simulink model "MAIN_Submitted_to_UMD_V2_PCLC_Sim_Hem"  (R2024a)
settings: Solver=ode3  StartTime=0.0  StopTime=T_end  FixedStep=0.01  RelTol=1e-3  EnableMultiTasking=on
values from neighbouring files (symbols this model uses):
  A1 = x(1)    [MAIN_Protocol_Simulation.m]    (also in find_fluid_profile.m)
  A2 = x(2)    [MAIN_Protocol_Simulation.m]    (also in find_fluid_profile.m)
  A3 = x(8)    [MAIN_Protocol_Simulation.m]    (also in find_fluid_profile.m)
  A4 = x(12)    [MAIN_Protocol_Simulation.m]    (also in find_fluid_profile.m)
  B_Gain = x(3)    [MAIN_Protocol_Simulation.m]    (also in find_fluid_profile.m)
  B_Loss = x(4)    [MAIN_Protocol_Simulation.m]    (also in find_fluid_profile.m)
  BP_Tar = x(14)    [MAIN_Protocol_Simulation.m]    (also in find_fluid_profile.m)
  BV0 = x(25)    [MAIN_Protocol_Simulation.m]    (also in find_fluid_profile.m)
  G1 = x(15)    [MAIN_Protocol_Simulation.m]    (also in find_fluid_profile.m)
  G2 = x(16)    [MAIN_Protocol_Simulation.m]    (also in find_fluid_profile.m)
  G3 = x(19)    [MAIN_Protocol_Simulation.m]    (also in find_fluid_profile.m)
  gap_btn_hem = 0.5    [find_fluid_profile.m]
  Gsv1 = x(6)    [MAIN_Protocol_Simulation.m]    (also in find_fluid_profile.m)
  Gsv2 = x(7)    [MAIN_Protocol_Simulation.m]    (also in find_fluid_profile.m)
  H = (0.04022*W-0.1436)/60    [find_fluid_profile.m]
  Hct0 = x(24)    [MAIN_Protocol_Simulation.m]    (also in find_fluid_profile.m)
  HR0 = x(22)    [MAIN_Protocol_Simulation.m]    (also in find_fluid_profile.m)
  Ki4 = x(21)    [MAIN_Protocol_Simulation.m]    (also in find_fluid_profile.m)
  Kp = x(5)    [MAIN_Protocol_Simulation.m]    (also in find_fluid_profile.m)
  Kp2 = x(10)    [MAIN_Protocol_Simulation.m]    (also in find_fluid_profile.m)
  Kp3 = x(11)    [MAIN_Protocol_Simulation.m]    (also in find_fluid_profile.m)
  Kp4 = x(20)    [MAIN_Protocol_Simulation.m]    (also in find_fluid_profile.m)
  maintain_time = 15    [find_fluid_profile.m]
  max_hem_time = 1    [find_fluid_profile.m]
  max_sim_time = 120    [find_fluid_profile.m]
  pow1 = x(17)    [MAIN_Protocol_Simulation.m]    (also in find_fluid_profile.m)
  pow2 = x(18)    [MAIN_Protocol_Simulation.m]    (also in find_fluid_profile.m)
  SV0 = x(23)    [MAIN_Protocol_Simulation.m]    (also in find_fluid_profile.m = theta_s(18))
  SV_Tar = x(9)    [MAIN_Protocol_Simulation.m]    (also in find_fluid_profile.m)
  TPR0 = x(13)    [MAIN_Protocol_Simulation.m]    (also in find_fluid_profile.m)
libraries: simulink x1
settings Model: Creator=Ramin  LastModifiedBy=yekanth
settings SolverCC: AlgebraicLoopSolver=TrustRegion
settings DataIOCC: LimitDataPoints=on  SaveFormat=Array  SignalLoggingSaveFormat=ModelDataLogs  ReturnWorkspaceOutputs=off
settings OptimizationCC: ExpressionDepthLimit=2147483647  LifeSpan=inf
settings DebuggingCC: UnderspecifiedInitializationDetection=Classic  MergeDetectMultiDrivingBlocksExec=none  SolverPrmCheckMsg=warning  FcnCallInpInsideContextMsg=warning  UnconnectedInputMsg=warning  UnconnectedOutputMsg=warning  UnconnectedLineMsg=warning  StateNameClashWarn=warning  SFUnexpectedBacktrackingDiag=warning  SFNoUnconditionalDefaultTransitionDiag=warning  SFExecutionAtInitializationDiag=none  ArithmeticOperatorsInVariantConditions=warning
settings HardwareCC: ProdBitPerPointer=32  ProdBitPerSizeT=32  ProdBitPerPtrDiffT=32  ProdLargestAtomicFloat=None  ProdIntDivRoundTo=Undefined  ProdEndianess=Unspecified  ProdWordSize=32  ProdHWDeviceType=32-bit Generic
settings ModelReferenceCC: EnableRefExpFcnMdlSchedulingChecks=on  PropagateSignalLabelsOutOfModel=off
settings SFSimCC: SimUseLocalCustomCode=off  LegacyBehaviorForPersistentVarInContinuousTime=on  CustomCodeUndefinedFunction=UseInterfaceOnly
settings RTWCC: RTWUseLocalCustomCode=off  GPUComputeCapability=3.5
settings CodeAppCC: StateflowObjectComments=on
settings GRTTargetCC: TargetLangStandard=C89/C90 (ANSI)
settings ConfigComp: CovMetricSettings=dw  CovSaveCumulativeToWorkspaceVar=on  CovSaveSingleToWorkspaceVar=on  CovExternalEMLEnable=off

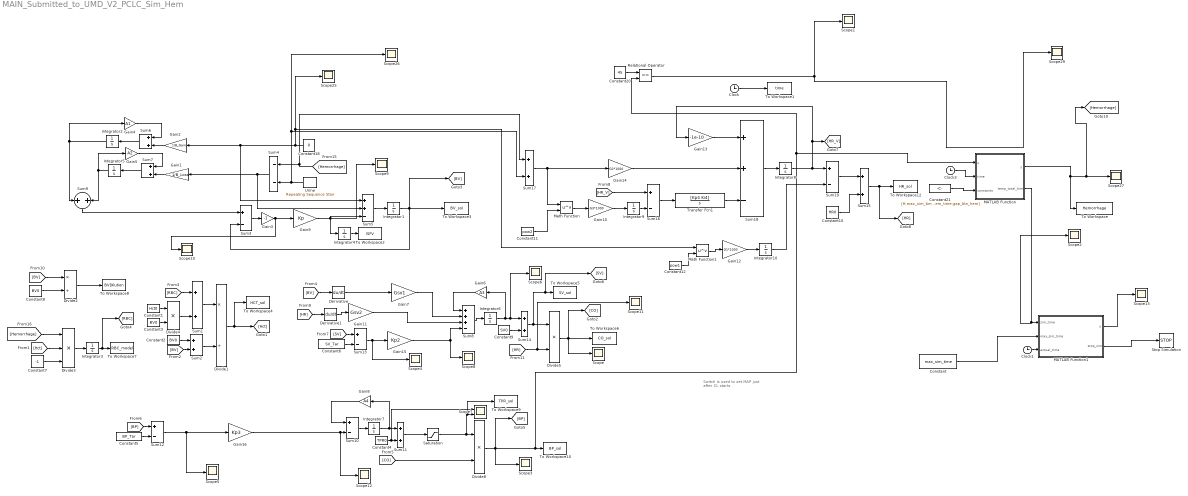
== system MAIN_Submitted_to_UMD_V2_PCLC_Sim_Hem ==
  note: Switch is used to set MAP just
      |  after CL starts
  Clock : Clock
  Clock1 : Clock
  Clock3 : Clock
  Constant : Constant  Value=max_sim_time
  Constant1 : Constant  Value=Hct0
  Constant10 : Constant  Value=HR0
  Constant11 : Constant  Value=pow2
  Constant12 : Constant  Value=pow1
  Constant18 : Constant  Value=0
  Constant2 : Constant  Value=BV0
  Constant20 : Constant  Value=45
  Constant21 : Constant  Value=[H;max_sim_time;maintain_time;max_hem_time;gap_btn_hem]  VectorParams1D=off
  Constant3 : Constant  Value=BV0
  Constant4 : Constant  Value=TPR0
  Constant5 : Constant  Value=BP_Tar
  Constant6 : Constant  Value=SV_Tar
  Constant7 : Constant  Value=-1
  Constant8 : Constant  Value=BV0
  Constant9 : Constant  Value=SV0
  Derivative : Derivative
  Derivative1 : Derivative
  Divide1 : Product  Inputs=*/
  Divide2 : Product  Inputs=*/
  Divide3 : Product  Inputs=***
  Divide4 : Product  Inputs=**
  Divide5 : Product  Inputs=**
  Divide8 : Product  Inputs=**
  Gain1 : Gain  Gain=1/B_Loss
  Gain10 : Gain  Gain=G3*1000
  Gain11 : Gain  Gain=Gsv2
  Gain12 : Gain  Gain=G1*1000
  Gain13 : Gain  Gain=-1e-10
  Gain14 : Gain  Gain=G2*1000
  Gain15 : Gain  Gain=Kp2
  Gain16 : Gain  Gain=Kp3
  Gain2 : Gain  Gain=1/B_Gain
  Gain3 : Gain  Gain=-1
  Gain4 : Gain  Gain=A1
  Gain5 : Gain  Gain=A2
  Gain6 : Gain  Gain=A3
  Gain7 : Gain  Gain=Gsv1
  Gain8 : Gain  Gain=A4
  Gain9 : Gain  Gain=Kp
  Integrator{1..10} (10 alike) : Integrator
  MATLAB Function : MATLAB Function  TreatAsAtomicUnit=on
  MATLAB Function1 : MATLAB Function  TreatAsAtomicUnit=on
  Math Function : Math  Operator=pow  SignedPower=on
  Math Function1 : Math  Operator=pow  SignedPower=on
  Relational Operator : RelationalOperator  Operator===  OutDataTypeStr=boolean  RndMeth=Simplest  InputSameDT=off
  Saturation : Saturate  UpperLimit=4000  LowerLimit=0
  Scope{,1..6,8..13,25..27,29} (17 alike) : Scope
  Scope7 : Scope  NumInputPorts=2
  Stop Simulation : Stop
  Sum{1..2,6..7,9,11,14..15,17} (9 alike) : Sum
  Sum{3,10,12..13,16,19} (6 alike) : Sum  Inputs=+-
  Sum18 : Sum  Inputs=++-
  Sum4 : Sum  Inputs=--
  Sum5 : Sum  Inputs=++-
  Sum8 : Sum  Inputs=+++-
  To Workspace : ToWorkspace  VariableName=Hemorrhage  SampleTime=-1
  To Workspace1 : ToWorkspace  VariableName=time  SampleTime=-1
  To Workspace10 : ToWorkspace  VariableName=BP_sol  SampleTime=-1
  To Workspace12 : ToWorkspace  VariableName=HR_sol  SampleTime=-1
  To Workspace2 : ToWorkspace  VariableName=ISFV  SampleTime=-1
  To Workspace3 : ToWorkspace  VariableName=BV_sol  SampleTime=-1
  To Workspace4 : ToWorkspace  VariableName=HCT_sol  SampleTime=-1
  To Workspace5 : ToWorkspace  VariableName=SV_sol  SampleTime=-1
  To Workspace6 : ToWorkspace  VariableName=CO_sol  SampleTime=-1
  To Workspace7 : ToWorkspace  VariableName=RBC_model  SampleTime=-1
  To Workspace8 : ToWorkspace  VariableName=BVDilution  SampleTime=-1
  To Workspace9 : ToWorkspace  VariableName=TPR_sol  SampleTime=-1
  Transfer Fcn1 : TransferFcn  Numerator=[Kp4 Ki4]  Denominator=[1 0]
  Urine : simulink/Sources/Repeating Sequence Stair  OutValues=Urine_inp  tsamp=SamplingTime  OutMin=[]  OutMax=[]  OutDataTypeStr=double  OutputDataTypeScalingMode=double  OutDataType=fixdt(0,8)  ConRadixGroup=Best Precision: Vector-wise  OutScaling=2^-12
  wires:
  Integrator4/1 -> To Workspace2/1
  Gain3/1 -> Gain9/1, Scope10/1
  Gain9/1 -> Scope9/1, Sum5/3, Integrator4/1
  Sum3/1 -> Gain3/1
  Sum5/1 -> Integrator1/1
  Divide3/1 -> Integrator3/1
  Integrator3/1 -> [RBC], To Workspace7/1
  [BV] -> Divide2/1
  Constant8/1 -> Divide2/2
  Divide2/1 -> To Workspace8/1
  [Hemorrhage] -> Divide3/1
  [Hct] -> Divide3/2
  Sum2/1 -> Divide1/2
  Constant7/1 -> Divide3/3
  Constant2/1 -> Sum2/1
  [BV] -> Sum2/2
  Constant1/1 -> Divide4/1
  Constant3/1 -> Divide4/2
  Divide4/1 -> Sum1/2
  [RBC] -> Sum1/1
  Sum1/1 -> Divide1/1
  Divide1/1 -> [Hct], To Workspace4/1
  Integrator2/1 -> Sum9/1, Gain4/1
  Sum6/1 -> Integrator2/1
  Gain4/1 -> Sum6/1
  Gain2/1 -> Sum6/2
  Integrator5/1 -> Sum9/2, Gain5/1
  Gain1/1 -> Sum7/2
  Sum7/1 -> Integrator5/1
  Gain5/1 -> Sum7/1
  Sum9/1 -> Sum3/1
  Integrator1/1 -> Sum3/2, To Workspace3/1, [BV]
  Gain7/1 -> Sum8/2
  Sum8/1 -> Integrator6/1
  Integrator6/1 -> Sum14/1, Scope6/1, Gain6/1
  Gain6/1 -> Sum8/1
  Constant9/1 -> Sum14/2
  Sum14/1 -> [SV], To Workspace5/1, Divide5/1
  Constant6/1 -> Sum13/2
  Sum13/1 -> Gain15/1, Scope4/1
  [SV] -> Sum13/1
  Gain15/1 -> Scope8/1, Sum8/4
  [BV] -> Derivative/1
  [HR] -> Scope11/1, Divide5/2
  [HR] -> Derivative1/1
  Gain11/1 -> Sum8/3
  Divide5/1 -> [CO], To Workspace6/1, Scope/1
  [BP] -> Sum12/1
  Gain8/1 -> Sum10/1
  Sum11/1 -> Saturation/1
  Sum10/1 -> Integrator7/1
  [CO] -> Divide8/2
  Sum12/1 -> Gain16/1, Scope5/1
  Constant5/1 -> Sum12/2
  Constant4/1 -> Scope7/1, Sum11/2
  Integrator7/1 -> Gain8/1, Sum11/1
  Derivative1/1 -> Gain11/1
  Derivative/1 -> Gain7/1
  Divide8/1 -> Relational Operator/2, MATLAB Function/1(u), To Workspace10/1, Scope3/1, [BP]
  Gain16/1 -> Scope12/1, Sum10/2
  Sum19/1 -> Sum15/1
  [HR_V] -> Sum16/1
  Sum4/1 -> Gain1/1, Sum5/2
  Gain12/1 -> Integrator10/1
  Integrator9/1 -> Sum16/2
  Constant11/1 -> Math Function/2
  Gain13/1 -> Sum18/1
  Math Function1/1 -> Gain12/1
  Constant18/1 -> Scope25/1, Math Function1/1, Sum5/1, Gain2/1
  Integrator8/1 -> [HR_V], Gain13/1, Sum19/1
  [Hemorrhage] -> Sum4/1, Sum17/1
  Gain14/1 -> Sum18/2
  Constant10/1 -> Sum15/2
  Urine/1 -> Scope26/1, Sum17/2, Sum4/2
  Integrator10/1 -> Sum19/2
  Sum15/1 -> [HR], To Workspace12/1
  Math Function/1 -> Gain10/1
  Gain10/1 -> Integrator9/1
  Sum18/1 -> Integrator8/1
  Transfer Fcn1/1 -> Sum18/3
  Sum16/1 -> Transfer Fcn1/1
  Constant12/1 -> Math Function1/2
  Sum17/1 -> Gain14/1, Math Function/1
  Saturation/1 -> To Workspace9/1, Scope7/2, Divide8/1
  Clock/1 -> To Workspace1/1
  Constant20/1 -> Relational Operator/1
  Constant21/1 -> MATLAB Function/3(constants)
  Relational Operator/1 -> Scope1/1, Scope29/1
  MATLAB Function/1(y) -> To Workspace/1, [Hemorrhage], Scope27/1
  MATLAB Function/2(temp_total_time) -> Scope2/1, MATLAB Function1/1(sim_time)
  Constant/1 -> MATLAB Function1/2(max_sim_time)
  Clock3/1 -> MATLAB Function/2(time)
  MATLAB Function1/1(y) -> Scope13/1
  MATLAB Function1/2(stop_sim) -> Stop Simulation/1
  Clock1/1 -> MATLAB Function1/3(actual_time)

== matlab function MAIN_Submitted_to_UMD_V2_PCLC_Sim_Hem/MATLAB Function1 ==
  data: sim_time input; max_sim_time input; y output; actual_time input; stop_sim output
function [y,stop_sim] = fcn(sim_time,max_sim_time,actual_time)

    persistent m

    if isempty(m)
        m = 0;
    end

    stop_sim = 0;

    if sim_time~=max_sim_time
        m = sim_time;
    end

    y = m;

    if (actual_time>10)&&(ceil(actual_time)==ceil(y))
        stop_sim = 1;
    end

== matlab function MAIN_Submitted_to_UMD_V2_PCLC_Sim_Hem/MATLAB Function ==
  data: u input; y output; time input; constants input; temp_total_time output
function [y,temp_total_time]  = fcn(u, time, constants)
    
    persistent m
    persistent n
    persistent hem_end_time
    persistent gap 
    persistent max_hem 
    persistent hem_triggered
    persistent total_time
    persistent triggered_end_time
    persistent k

    %Constants (Extract all constants)
    H = constants(1);
    max_sim_time = constants(2);
    maintain_time = constants(3);
    max_hem_time = constants(4);
    gap_btn_hem = constants(5);

    if isempty(m)
        m = 1;
        
    end

    if isempty(total_time)
        total_time = max_sim_time;
    end

    if isempty(k)
        k = 0;
    end

    if isempty(n)
        n = 0;
    end

    if isempty(hem_end_time)
        hem_end_time = max_sim_time;
    end

    if isempty(hem_triggered)
        hem_triggered = -3;
    end

    if isempty(triggered_end_time)
        triggered_end_time = -5;
    end

    if isempty(gap)
        gap = 0;
    end

    if isempty(max_hem)
        max_hem = 0;
    end

    %Initialize Hemorrhage and BP in each iteration

    y = 0;
    BP = u;
    
    temp_total_time = max_sim_time;

    % If BP goes below 45 for first time, end hemorrhage

    if (BP<=45)&&(m==1)
        m = 0;
        hem_end_time = time;
        total_time = hem_end_time+maintain_time;
        temp_total_time = total_time;
    end

    if (BP>45)&&(time<hem_end_time)
        y = m*H;
    end

    % Keep Simulating Hemorrhage until the first time hemorrhage ends and
    % maintain time
    if (time<hem_end_time+maintain_time)&&(time>hem_end_time)&&(BP>48)

        %Calculate gap between two hemorrhages 
        if (k==0)
            gap = hem_triggered - triggered_end_time;
        end

        n = 1;
        hem_triggered = time;
        
         
    end

    % Keep Simulating each triggered hemorrhage for a minute

    if (time<hem_triggered+max_hem_time)&&(gap>gap_btn_hem)
        y = n*H;
        triggered_end_time = time;
        k = 1;
    else
        k = 0;
    end
